simulink model "VDC25_old"  (R2022a)
settings: Solver=FixedStepAuto  StartTime=0.0  StopTime=10.0  FixedStep=vdc_TimeStep  RelTol=1e-3
undefined symbols (not defined in the file): param, param_vdc
settings Model: Creator=jutri  LastModifiedBy=Usuario
settings ModelReferenceCC: EnableRefExpFcnMdlSchedulingChecks=off
settings RTWCC: Description=Generic Real-Time Target  GPUComputeCapability=5.0

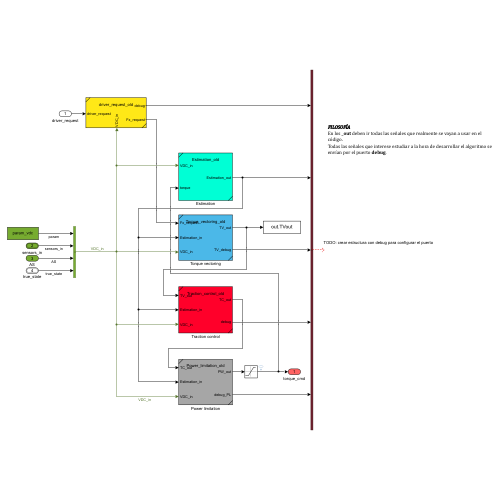
[thumbnail: Simulink's stored preview of the top-level diagram]
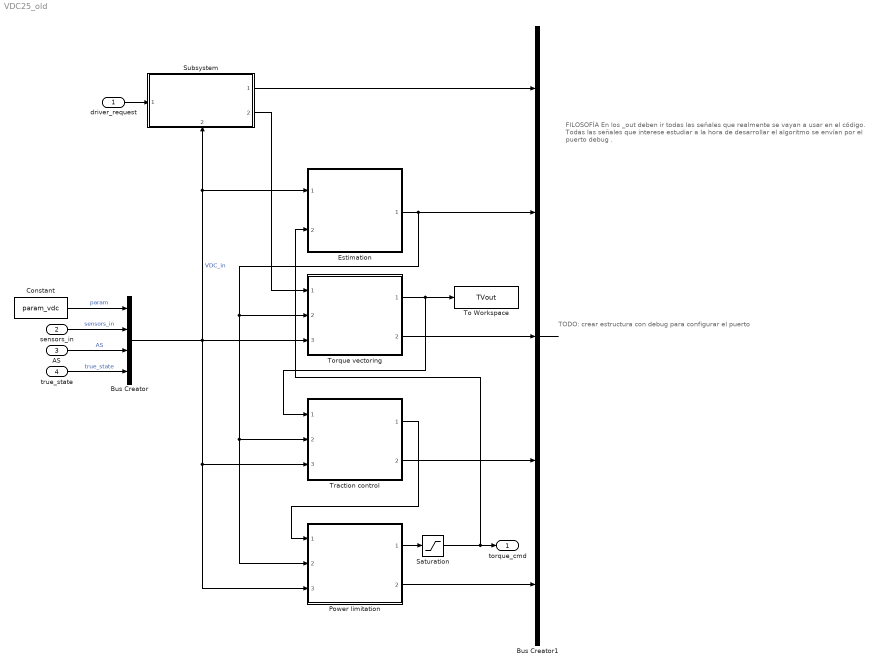
== system VDC25_old ==
  note: TODO: crear estructura con debug para configurar el puerto
  note: FILOSOFÍA
      | En los _out deben ir todas las señales que realmente se vayan a usar en el código.
      | Todas las señales que interese estudiar a la hora de desarrollar el algoritmo se envían por el puerto debug .
  driver_request : Inport
  sensors_in : Inport  Port=2  OutDataTypeStr=Bus: sensorBus
  AS : Inport  Port=3
  true_state : Inport  Port=4  OutDataTypeStr=Bus: stateBus
  Bus Creator : BusCreator  Inputs=4
  Bus Creator1 : BusCreator  Inputs=5
  Constant : Constant  Value=param_vdc  OutDataTypeStr=Bus: vdcBus
  Estimation : Subsystem  ReferencedSubsystem=Estimation_old
  Power limitation : Subsystem  ReferencedSubsystem=Power_limitation_old
  Saturation : Saturate  UpperLimit=param.torque_limit_positive  LowerLimit=param.torque_limit_negative
  Subsystem : Subsystem  ReferencedSubsystem=driver_request_old
      settings: PortSchema="{\"entries\":[{\"content\":{\"sides\":[{\"content\":{\"connectorIds\":[\"In1\"]},\"type\":\"ConnectorPlacement.EquallySpacedRectSide\",\"uuid\":\"6d0b78b3-ffc0-496d-8d3a-7ba3f556f803\"},{\"content\":{\"connectorIds\":[\"Out1\",\"Out2\"],\"side\":\"RIGHT\"},\"type\":\"ConnectorPlacement.EquallySpacedRectSide\",\"uuid\":\"be1dfba9-3592-437e-9363-a3609142bbc4\"},{\"content\":{\"connectorIds\":[],\"side\":\"TOP\"},\"type\":\"ConnectorPlacement.EquallySpacedRectSide\",\"uuid\":\"ddffd853-c46f-4213-b654-9451d95e6853\"},{\"content\":{\"connectorIds\":[\"In2\"],\"side\":\"BOTTOM\"},\"type\":\"ConnectorPlacement.EquallySpacedRectSide\",\"uuid\":\"b463dc20-ae30-4837-a1c3-1d0c4501f548\"}]},\"type\":\"ConnectorPlacement.EquallySpacedConnector\",\"uuid\":\"75a8dd9f-93ed-4a7a-b725-fd6938405663\"}],\"packageUris\":[\"http://schema.mathworks.com/mf0/Connector/R2020b\"],\"version\":\"1.0\"}"
  To Workspace : ToWorkspace  VariableName=TVout  SaveFormat=Timeseries  SampleTime=-1
  Torque vectoring : Subsystem  ReferencedSubsystem=Torque_vectoring_old
  Traction control : Subsystem  ReferencedSubsystem=Traction_control_old
  torque_cmd : Outport
  wires:
  driver_request/1 -> Subsystem/1
  Bus Creator/1 -> Power limitation/3, Traction control/3, Subsystem/2, Estimation/1, Torque vectoring/3  "VDC_in"
  Constant/1 -> Bus Creator/1  "param"
  sensors_in/1 -> Bus Creator/2  "sensors_in"
  AS/1 -> Bus Creator/3  "AS"
  Torque vectoring/1 -> To Workspace/1, Traction control/1
  Traction control/1 -> Power limitation/1
  Subsystem/2 -> Torque vectoring/1
  Subsystem/1 -> Bus Creator1/1
  Estimation/1 -> Torque vectoring/2, Traction control/2, Power limitation/2, Bus Creator1/2
  Torque vectoring/2 -> Bus Creator1/3
  Traction control/2 -> Bus Creator1/4
  Power limitation/2 -> Bus Creator1/5
  Power limitation/1 -> Saturation/1
  true_state/1 -> Bus Creator/4  "true_state"
  Bus Creator1/1 -> ?
  Saturation/1 -> torque_cmd/1, Estimation/2
